simulink model "TweeprSystem"  (R2021a)
settings: Solver=VariableStepAuto  StartTime=0.0  StopTime=10.0  RelTol=1e-3
values from neighbouring files (symbols this model uses):
  A = [0,         0,                  1,                  0 ... (first row only)    [TweeprConfig.m]
  B = [0;        0;                 1/mb;              1/(L*mb)]    [TweeprConfig.m]
  K = lqr(A, B, Q, R)    [TweeprConfig.m]
undefined symbols (not defined in the file or in its folder): x0
settings Model: Creator=ssant  LastModifiedBy=ssant

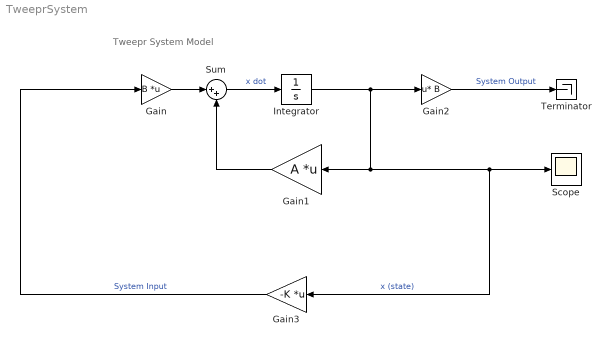
== system TweeprSystem ==
  note: Tweepr System Model
  Gain : Gain  Gain=B  Multiplication=Matrix(K*u)
  Gain1 : Gain  Gain=A  Multiplication=Matrix(K*u) (u vector)
  Gain2 : Gain  Gain=B  Multiplication=Matrix(u*K)
  Gain3 : Gain  Gain=-K  Multiplication=Matrix(K*u)
  Integrator : Integrator  InitialCondition=x0
  Scope : Scope
  Sum : Sum  Inputs=|++
  Terminator : Terminator
  wires:
  Gain/1 -> Sum/1
  Sum/1 -> Integrator/1  "x dot"
  Gain1/1 -> Sum/2
  Integrator/1 -> Gain2/1, Scope/1, Gain3/1, Gain1/1  "x (state)"
  Gain3/1 -> Gain/1  "System Input"
  Gain2/1 -> Terminator/1  "System Output"
